simulink model "hdl_generation_2"  (R2024b)
settings: Solver=VariableStepAuto  StartTime=0.0  StopTime=10.0  RelTol=1e-3
libraries: matrix_library x2, slpidlib x1, aerolibutil x1
settings Model: Creator=keybo  LastModifiedBy=keybo

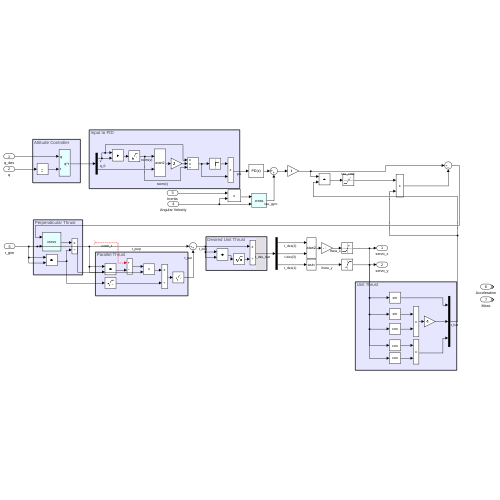
[thumbnail: Simulink's stored preview of the top-level diagram]
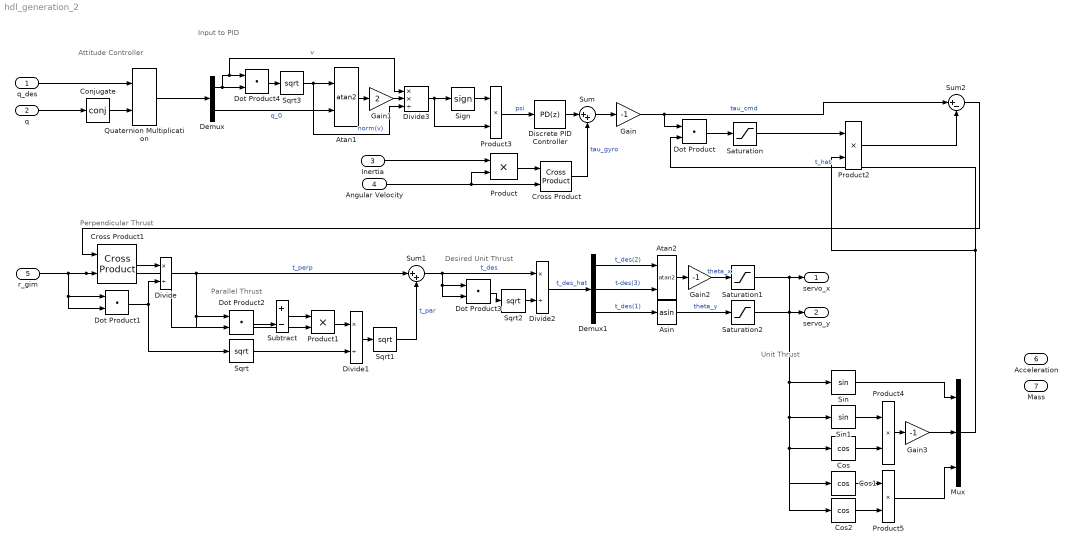
== system hdl_generation_2 ==
  note: Unit Thrust
  note: Input to PID
  note: Desired Unit Thrust
  note: Parallel Thrust
  note: Perpendicular Thrust
  note: Attitude Controller
  q_des : Inport  PortDimensions=4
  q : Inport  Port=2  PortDimensions=4
  Inertia : Inport  Port=3
  Angular Velocity : Inport  Port=4
  r_gim : Inport  Port=5
  Acceleration : Inport  Port=6
  Mass : Inport  Port=7
  Asin : Trigonometry  Operator=asin
  Atan1 : Trigonometry  Operator=atan2
  Atan2 : Trigonometry  Operator=atan2
  Conjugate : Math  Operator=conj  SignedPower=on  RndMeth=Zero
  Cos : Trigonometry  Operator=cos
  Cos1 : Trigonometry  Operator=cos
  Cos2 : Trigonometry  Operator=cos
  Cross Product : matrix_library/Cross Product
  Cross Product1 : matrix_library/Cross Product
  Demux : Demux  Outputs=2
  Demux1 : Demux  Outputs=3
  Discrete PID Controller : slpidlib/PID Controller  Controller=PD  Form=Parallel  TimeDomain=Discrete-time  UseExternalTs=off  SampleTime=0.001  IntegratorMethod=Forward Euler  FilterMethod=Forward Euler  ControllerParametersSource=internal  P=1  I=1  UseKiTs=off  D=1  UseExternalDerivativeSource=off  N=1  UseFilter=on  TunerSelectOption=Transfer Function Based (PID Tuner App)  InitialConditionSource=internal  InitialConditionForIntegrator=0  InitialConditionForFilter=0  DifferentiatorICPrevScaledInput=0  ExternalReset=none  TrackingMode=off  Kt=1  LimitOutput=off  SatLimitsSource=internal  UpperSaturationLimit=inf  LowerSaturationLimit=-inf  LinearizeAsGain=off  AntiWindupMode=none  Kb=1  LimitIntegrator=off  UpperIntegratorSaturationLimit=inf  LowerIntegratorSaturationLimit=-inf  POutMin=[]  POutMax=[]  IOutMin=[]  IOutMax=[]  DOutMin=[]  DOutMax=[]  NOutMin=[]  NOutMax=[]  SumOutMin=[]  SumOutMax=[]  SaturationOutMin=[]  SaturationOutMax=[]  PParamMin=[]  PParamMax=[]  IParamMin=[]  IParamMax=[]  DParamMin=[]  DParamMax=[]  NParamMin=[]  NParamMax=[]  KbParamMin=[]  KbParamMax=[]  KtParamMin=[]  KtParamMax=[]  KbOutMin=[]  KbOutMax=[]  KtOutMin=[]  KtOutMax=[]  IntegratorOutMin=[]  IntegratorOutMax=[]  FilterOutMin=[]  FilterOutMax=[]  SumI1OutMin=[]  SumI1OutMax=[]  SumI2OutMin=[]  SumI2OutMax=[]  SumI3OutMin=[]  SumI3OutMax=[]  SumI4OutMin=[]  SumI4OutMax=[]  SumDOutMin=[]  SumDOutMax=[]  DifferentiatorOutMin=[]  DifferentiatorOutMax=[]  FilterDiffOutCoefMin=[]  FilterDiffOutCoefMax=[]  ReciprocalOutMin=[]  ReciprocalOutMax=[]  SumDenOutMin=[]  SumDenOutMax=[]  SumNumOutMin=[]  SumNumOutMax=[]  DivideOutMin=[]  DivideOutMax=[]  UdiffTsProdOutMin=[]  UdiffTsProdOutMax=[]  NTsProdOutMin=[]  NTsProdOutMax=[]  UintegralTsProdOutMin=[]  UintegralTsProdOutMax=[]  UngainTsProdOutMin=[]  UngainTsProdOutMax=[]  ClampingZeroOutDataTypeStr=Inherit: Inherit via back propagation  ClampingZeroOutMin=[]  ClampingZeroOutMax=[]  FilterDenConstantOutDataTypeStr=Inherit: Inherit via back propagation  FilterDenConstantOutMin=[]  FilterDenConstantOutMax=[]  PCopyOutDataTypeStr=Inherit: Inherit via back propagation  PCopyOutMin=[]  PCopyOutMax=[]  NCopyOutDataTypeStr=Inherit: Inherit via back propagation  NCopyOutMin=[]  NCopyOutMax=[]  IntegratorContinuousStateAttributes=''  IntegratorStateMustResolveToSignalObject=off  IntegratorRTWStateStorageClass=Auto  FilterContinuousStateAttributes=''  FilterStateMustResolveToSignalObject=off  FilterRTWStateStorageClass=Auto  ParallelPVariant=InternalParameters  IdealPVariant=Disabled  IVariant=Disabled  DVariant=InternalParameters  IntegratorVariant=Disabled  SatVariant=Disabled  AWVariant=Disabled  PCopyVariant=Disabled  TRVariant=Disabled  FdbkBlocksVariant=Forward  IdealPFdbkVariant=Disabled  SatFdbkVariant=Disabled  DerivativeFilterVariant=ForwardEulerFilter  NVariant=InternalParameters  NCopyVariant=Disabled  FilterICVariant=InternalICsFilter  IntegratorICVariant=Disabled  ExternalResetVariant=Disabled  TRSumVariant=Passthrough  SumFdbkVariant=Disabled  SumVariant=Sum_PD  TsampFilterVariant=InternalTs  TsampNgainVariant=Passthrough  TsampIntegralVariant=Disabled_SignalSpec  ExternalSaturationOutDataTypeStr=Inherit: Same as second input  DerivativeSourceVariant=ErrorSignal  PreIntVariant=InternalPreInt
      settings: LibrarySourceBlock=simulink/Discrete/Discrete PID Controller
  Divide : Product  Inputs=*/
  Divide1 : Product  Inputs=*/
  Divide2 : Product  Inputs=*/
  Divide3 : Product  Inputs=**/
  Dot Product{,1..4} (5 alike) : DotProduct  OutDataTypeStr=Inherit: Inherit via internal rule
  Gain : Gain  Gain=-1
  Gain1 : Gain  Gain=2
  Gain2 : Gain  Gain=-1
  Gain3 : Gain  Gain=-1
  Mux : Mux  Inputs=3
  Product{,1..5} (6 alike) : Product
  Quaternion Multiplication : aerolibutil/Quaternion Multiplication
  Saturation : Saturate
  Saturation1 : Saturate
  Saturation2 : Saturate
  Sign : Signum
  Sin : Trigonometry
  Sin1 : Trigonometry
  Sqrt{,1..3} (4 alike) : Sqrt
  Subtract : Sum  Inputs=+-
  Sum : Sum  Inputs=|++
  Sum1 : Sum  Inputs=|++
  Sum2 : Sum  Inputs=|+-
  servo_x : Outport  VectorParamsAs1DForOutWhenUnconnected=off
  servo_y : Outport  Port=2  VectorParamsAs1DForOutWhenUnconnected=off
  wires:
  q/1 -> Conjugate/1
  q_des/1 -> Quaternion Multiplication/1
  Conjugate/1 -> Quaternion Multiplication/2
  Discrete PID Controller/1 -> Sum/1
  Inertia/1 -> Product/1
  Angular Velocity/1 -> Product/2, Cross Product/2
  Product/1 -> Cross Product/1
  Cross Product/1 -> Sum/2  "tau_gyro"
  Gain/1 -> Sum2/1, Dot Product/1  "tau_cmd"
  Dot Product/1 -> Saturation/1
  Sum2/1 -> Cross Product1/1
  Cross Product1/1 -> Divide/1
  Divide/1 -> Dot Product2/2, Dot Product2/1, Sum1/1  "t_perp"
  ? -> Subtract/1  "norm_t"
  Dot Product1/1 -> Sqrt/1, Divide/2
  Sqrt1/1 -> Sum1/2  "t_par"
  r_gim/1 -> Dot Product1/1, Dot Product1/2, Product1/2, Cross Product1/2
  Divide1/1 -> Sqrt1/1
  Sqrt/1 -> Divide1/2
  Product1/1 -> Divide1/1
  Subtract/1 -> Product1/1
  Dot Product2/1 -> Subtract/2
  Atan2/1 -> Gain2/1
  Asin/1 -> Saturation2/1  "theta_y"
  Sum/1 -> Gain/1
  Saturation/1 -> Product2/1
  Product2/1 -> Sum2/2
  Sum1/1 -> Dot Product3/1, Dot Product3/2, Divide2/1  "t_des"
  Divide2/1 -> Demux1/1  "t_des_hat"
  Dot Product3/1 -> Sqrt2/1
  Sqrt2/1 -> Divide2/2
  Demux1/3 -> Asin/1  "t_des(1)"
  Demux1/2 -> Atan2/2  "t-des(3)"
  Demux1/1 -> Atan2/1  "t_des(2)"
  Product3/1 -> Discrete PID Controller/1  "psi"
  Demux/1 -> Dot Product4/2, Divide3/1, Dot Product4/1  "v"
  Divide3/1 -> Product3/2, Sign/1
  Demux/2 -> Atan1/2  "q_0"
  Sqrt3/1 -> Divide3/3, Atan1/1  "norm(v)"
  Dot Product4/1 -> Sqrt3/1
  Sign/1 -> Product3/1
  Quaternion Multiplication/1 -> Demux/1
  Gain1/1 -> Divide3/2
  Atan1/1 -> Gain1/1
  Gain2/1 -> Saturation1/1  "theta_x"
  Saturation1/1 -> Sin1/1, Cos1/1, servo_x/1
  Saturation2/1 -> Cos/1, Cos2/1, Sin/1, servo_y/1
  Product5/1 -> Mux/3
  Product4/1 -> Gain3/1
  Cos/1 -> Product4/2
  Cos2/1 -> Product5/2
  Sin/1 -> Mux/1
  Gain3/1 -> Mux/2
  Cos1/1 -> Product5/1
  Mux/1 -> Dot Product/2, Product2/2  "t_hat"
  Sin1/1 -> Product4/1
